simulink model "BruceMotor"  (R2024b)
settings: Solver=VariableStepAuto  StartTime=0.0  StopTime=2  RelTol=1e-3
InitFcn:
  | MotorSimulationParams
values from neighbouring files (symbols this model uses):
  B_PMSM = 0    [MotorSimulationParams.m]
  F_PMSM = 1e-3    (= 0.001)    [MotorSimulationParams.m]
  Id_D = 0    [MotorSimulationParams.m]
  Id_I = 0    [MotorSimulationParams.m]
  Id_P = 10    [MotorSimulationParams.m]
  Id_ref = 0    [MotorSimulationParams.m]
  Iq_D = 0    [MotorSimulationParams.m]
  Iq_I = 0    [MotorSimulationParams.m]
  Iq_P = 100    [MotorSimulationParams.m]
  J_PMSM = 1.879e-6    (= 1.879e-06)    [MotorSimulationParams.m]
  Load_Torque = 0    [MotorSimulationParams.m]
  Pole_Pairs = 1    [MotorSimulationParams.m]
  Ref_Torque = 1e-5    (= 1e-05)    [MotorSimulationParams.m]
  Rline = 1e-3    (= 0.001)    [MotorSimulationParams.m]
  Rs = 312e-3    (= 0.312)    [MotorSimulationParams.m]
  Speed_D = 0    [MotorSimulationParams.m]
  Speed_I = 0    [MotorSimulationParams.m]
  Speed_P = 100    [MotorSimulationParams.m]
  Speed_Ref = Wrated    (= 282.743338823)    [MotorSimulationParams.m]
  Tstep = 5e-6    (= 5e-06)    [MotorSimulationParams.m]
libraries: spsHalfBridgeConverterLib x3, spsdq0toabcLib x2, spsDCVoltageSourceLib x1, spsPermanentMagnetSynchronousMachineLib x1, simulink x1, spsThreePhaseParallelRLCBranchLib x1, spsabctodq0Lib x1, spspowerguiLib x1
settings Model: Creator=pickl  LastModifiedBy=pickl
settings SolverCC: ZeroCrossAlgorithm=Adaptive
settings DebuggingCC: MaskedZcDiagnostic=none  IgnoredZcDiagnostic=none

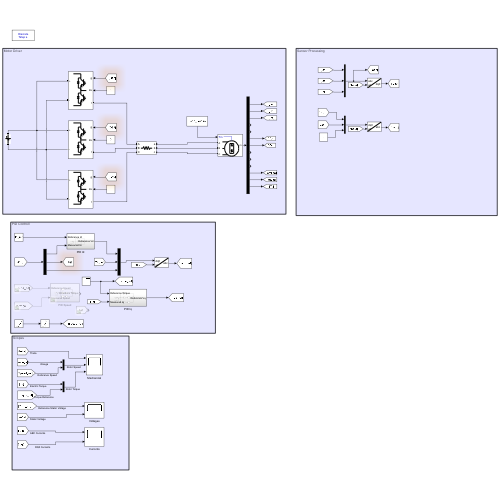
[thumbnail: Simulink's stored preview of the top-level diagram]
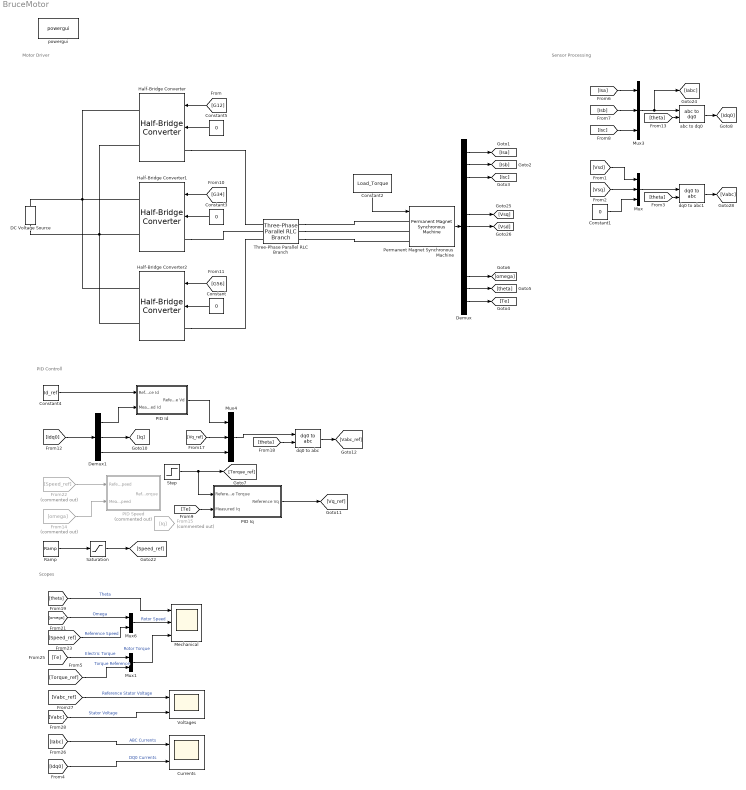
== system BruceMotor ==
  note: Scopes
  note: PID Controll
  note: Sensor Processing
  note: Motor Driver
  Constant{,1,3,5} (4 alike) : Constant  Value=0
  Constant2 : Constant  Value=Load_Torque
  Constant4 : Constant  Value=Id_ref
  Currents : Scope  NumInputPorts=2
  DC Voltage Source : spsDCVoltageSourceLib/DC Voltage Source  Amplitude=10  Measurements=None
  Demux : Demux  Outputs=13
  Demux1 : Demux  Outputs=3
  From14 : From  Commented=on  GotoTag=omega
  From15 : From  Commented=on  GotoTag=Iq
  From22 : From  Commented=on  GotoTag=Speed_ref
  Half-Bridge Converter : spsHalfBridgeConverterLib/Half-Bridge Converter  ModelType=Switching devices  Ron=1e-3  Rs=1e6  Cs=inf  Vforward=[0,0]  Ron_Diode=1e-3  Rs_Diode=1e6  Cs_Diode=inf  Vf_Diode=1e-3  Rs_CurrentSource=inf  Ron_ACsource=1e-3
      settings: LibrarySourceBlock=sps_lib/Power Electronics/Half-Bridge Converter
  Half-Bridge Converter1 : spsHalfBridgeConverterLib/Half-Bridge Converter  ModelType=Switching devices  Ron=1e-3  Rs=1e6  Cs=inf  Vforward=[0,0]  Ron_Diode=1e-3  Rs_Diode=1e6  Cs_Diode=inf  Vf_Diode=1e-3  Rs_CurrentSource=inf  Ron_ACsource=1e-3
      settings: LibrarySourceBlock=sps_lib/Power Electronics/Half-Bridge Converter
  Half-Bridge Converter2 : spsHalfBridgeConverterLib/Half-Bridge Converter  ModelType=Switching devices  Ron=1e-3  Rs=1e6  Cs=inf  Vforward=[0,0]  Ron_Diode=1e-3  Rs_Diode=1e6  Cs_Diode=inf  Vf_Diode=1e-3  Rs_CurrentSource=inf  Ron_ACsource=1e-3
      settings: LibrarySourceBlock=sps_lib/Power Electronics/Half-Bridge Converter
  Mechanical : Scope  NumInputPorts=3
  Mux : Mux  Inputs=3
  Mux1 : Mux  Inputs=2
  Mux3 : Mux  Inputs=3
  Mux4 : Mux  Inputs=3
  Mux6 : Mux  Inputs=2
  PID Id : Subsystem
  PID Iq : Subsystem
  PID Speed : Subsystem  Commented=on
  Permanent Magnet Synchronous Machine : spsPermanentMagnetSynchronousMachineLib/Permanent Magnet Synchronous Machine  NbPhases=3  FluxDistribution=Sinusoidal  RotorType=Round  MechanicalLoad=Torque Tm  PresetModel=No  ShowDetailedParameters=on  MeasurementBus=off  Resistance=Rs  Inductance=8.5e-3  dqInductances=[8.5e-3,8.5e-3]  La=Lq  MachineConstant=Voltage Constant (V_peak L-L / krpm)  Flux=0.0091888  VoltageCst=Kv  TorqueCst=0.04135  Flat=120  Mechanical=[J_PMSM, F_PMSM, Pole_Pairs, B_PMSM]  PolePairs=4  InitialConditions=[0,0, 0,0]  InitialConditions5ph=[0 0 0 0 0 0]  RefAngle=Aligned with phase A axis (original Park)  IterativeDiscreteModel=Trapezoidal non iterative  TsBlock=-1  TsPowergui=0
  Ramp : simulink/Sources/Ramp  slope=Wrated/Tramp  start=0.5  InitialOutput=0
  Saturation : Saturate  UpperLimit=Speed_Ref  LowerLimit=-Speed_Ref
  Step : Step  Time=0.2  After=Ref_Torque  SampleTime=0
  Three-Phase Parallel RLC Branch : spsThreePhaseParallelRLCBranchLib/Three-Phase Parallel RLC Branch  LConnTagsString=A|B|C  RConnTagsString=A|B|C  BranchType=R  Resistance=Rline  Inductance=1e-3  Capacitance=1e-6  Measurements=None
  Voltages : Scope  NumInputPorts=2
  abc to dq0 : spsabctodq0Lib/abc to dq0  Alignment=Aligned with phase A axis
  dq0 to abc : spsdq0toabcLib/dq0 to abc  Alignment=Aligned with phase A axis
  dq0 to abc1 : spsdq0toabcLib/dq0 to abc  Alignment=Aligned with phase A axis
  powergui : spspowerguiLib/powergui  Priority=1  SimulationMode=Discrete  SampleTime=Tstep  frequency=60  Iterations=50  frequencyindice=0  Pbase=100e6  ErrMax=1e-4  UnitsV=kV  UnitsW=MW  buscounter=0  FunctionMessages=off  echomessages=off  EnableUseOfTLC=off  CurrentSourceSwitches=off  DisableSnubberDevices=off  DisableRonSwitches=off  DisableVfSwitches=off  DisplayEquations=off  AutomaticDiscreteSolvers=off  SolverType=Tustin/Backward Euler (TBE)  Interpol=off  ExternalGateDelay=off  methode=off  Ts=100  x0status=zero  SPID=on  SwTol=0  HookPort=off  NonlinearTolerance=1e-4  nMaxIteration=100  ContinueOnMaxIteration=off  RestoreLinks=warning  ResistiveCurrentMeasurement=off  Frange=[0:2:500]  Ylog=off  Xlog=on  ShowGrid=off  save=off  variable=ZData  structure=0  ZoomFFT=off  StartTime=0.0  cycles=1  DisplayStyle=1  fundamental=60  FreqAxis=off  MaxFrequency=1000  frequencyindicesteady=1  RmsSteady=1  display=off
  wires:
  Permanent Magnet Synchronous Machine/1 -> Demux/1
  Demux/1 -> [Isa]
  Demux/2 -> [Isb]
  Demux/3 -> [Isc]
  [Isa] -> Mux3/1
  [Isb] -> Mux3/2
  [Isc] -> Mux3/3
  Mux3/1 -> [Iabc], abc to dq0/1
  abc to dq0/1 -> [Idq0]
  [Idq0] -> Demux1/1
  Demux1/3 -> Mux4/3
  Demux1/2 -> [Iq]
  [Vq_ref] -> Mux4/2
  Mux4/1 -> dq0 to abc/1
  [theta] -> abc to dq0/2
  [theta] -> dq0 to abc/2
  dq0 to abc/1 -> [Vabc_ref]
  [theta] -> Mechanical/1  "Theta"
  [omega] -> Mux6/1  "Omega"
  [Speed_ref] -> Mux6/2  "Reference Speed"
  Mux6/1 -> Mechanical/2  "Rotor Speed"
  Ramp/1 -> Saturation/1
  Saturation/1 -> [Speed_ref]
  [Vsd] -> Mux/1
  [Vsq] -> Mux/2
  Constant1/1 -> Mux/3
  Demux/6 -> [Vsq]
  Demux/7 -> [Vsd]
  Demux/13 -> [Te]
  Demux/12 -> [theta]
  Demux/11 -> [omega]
  Mux/1 -> dq0 to abc1/1
  dq0 to abc1/1 -> [Vabc]
  [theta] -> dq0 to abc1/2
  Constant2/1 -> Permanent Magnet Synchronous Machine/1
  PID Iq/1(Reference Vq) -> [Vq_ref]
  From22/1 -> PID Speed/1(Reference Speed)
  From14/1 -> PID Speed/2(Measured Speed)
  Demux1/1 -> PID Id/2(Measured Id)
  Constant4/1 -> PID Id/1(Reference Id)
  PID Id/1(Reference Vd) -> Mux4/1
  [Vabc_ref] -> Voltages/1  "Reference Stator Voltage"
  [Vabc] -> Voltages/2  "Stator Voltage"
  [Iabc] -> Currents/1  "ABC Currents"
  [Idq0] -> Currents/2  "DQ0 Currents"
  Step/1 -> PID Iq/1(Reference Torque), [Torque_ref]
  [Te] -> Mux1/1  "Electric Torque"
  [Torque_ref] -> Mux1/2  "Torque Reference"
  Mux1/1 -> Mechanical/3  "Rotor Torque"
  [Te] -> PID Iq/2(Measured Iq)
  [G34] -> Half-Bridge Converter1/1
  Constant/1 -> Half-Bridge Converter2/2
  [G56] -> Half-Bridge Converter2/1
  [G12] -> Half-Bridge Converter/1
  Constant3/1 -> Half-Bridge Converter1/2
  Constant5/1 -> Half-Bridge Converter/2
  connections:
  Three-Phase Parallel RLC Branch/RConn2 -- Permanent Magnet Synchronous Machine/LConn2
  Three-Phase Parallel RLC Branch/RConn1 -- Permanent Magnet Synchronous Machine/LConn1
  Three-Phase Parallel RLC Branch/RConn3 -- Permanent Magnet Synchronous Machine/LConn3
  Half-Bridge Converter1/RConn1 -- DC Voltage Source/RConn1 -- Half-Bridge Converter2/RConn1 -- Half-Bridge Converter/RConn1
  DC Voltage Source/LConn1 -- Half-Bridge Converter/RConn2 -- Half-Bridge Converter2/RConn2 -- Half-Bridge Converter1/RConn2
  Half-Bridge Converter/LConn1 -- Three-Phase Parallel RLC Branch/LConn1
  Half-Bridge Converter1/LConn1 -- Three-Phase Parallel RLC Branch/LConn2
  Half-Bridge Converter2/LConn1 -- Three-Phase Parallel RLC Branch/LConn3

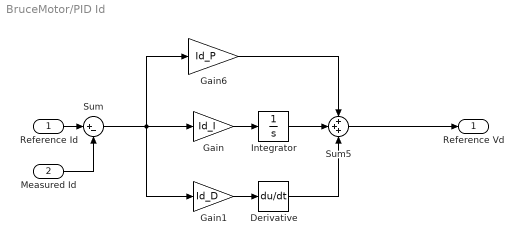
== system BruceMotor/PID Id ==
  Reference Id : Inport
  Measured Id : Inport  Port=2
  Derivative : Derivative
  Gain : Gain  Gain=Id_I
  Gain1 : Gain  Gain=Id_D
  Gain6 : Gain  Gain=Id_P
  Integrator : Integrator
  Sum : Sum  Inputs=|+-
  Sum5 : Sum  Inputs=+++
  Reference Vd : Outport
  wires:
  Reference Id/1 -> Sum/1
  Measured Id/1 -> Sum/2
  Gain/1 -> Integrator/1
  Gain6/1 -> Sum5/1
  Sum/1 -> Gain1/1, Gain6/1, Gain/1
  Gain1/1 -> Derivative/1
  Sum5/1 -> Reference Vd/1
  Integrator/1 -> Sum5/2
  Derivative/1 -> Sum5/3

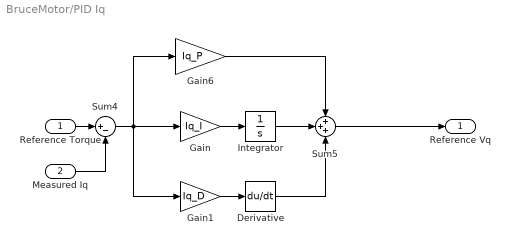
== system BruceMotor/PID Iq ==
  Reference Torque : Inport
  Measured Iq : Inport  Port=2
  Derivative : Derivative
  Gain : Gain  Gain=Iq_I
  Gain1 : Gain  Gain=Iq_D
  Gain6 : Gain  Gain=Iq_P
  Integrator : Integrator
  Sum4 : Sum  Inputs=|+-
  Sum5 : Sum  Inputs=+++
  Reference Vq : Outport
  wires:
  Measured Iq/1 -> Sum4/2
  Derivative/1 -> Sum5/3
  Gain/1 -> Integrator/1
  Sum4/1 -> Gain1/1, Gain6/1, Gain/1
  Gain6/1 -> Sum5/1
  Reference Torque/1 -> Sum4/1
  Sum5/1 -> Reference Vq/1
  Integrator/1 -> Sum5/2
  Gain1/1 -> Derivative/1

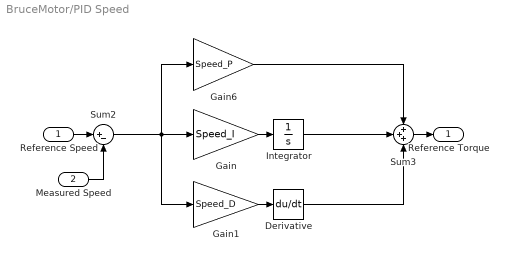
== system BruceMotor/PID Speed ==
  Reference Speed : Inport
  Measured Speed : Inport  Port=2
  Derivative : Derivative
  Gain : Gain  Gain=Speed_I
  Gain1 : Gain  Gain=Speed_D
  Gain6 : Gain  Gain=Speed_P
  Integrator : Integrator
  Sum2 : Sum  Inputs=|+-
  Sum3 : Sum  Inputs=+++
  Reference Torque : Outport
  wires:
  Sum3/1 -> Reference Torque/1
  Derivative/1 -> Sum3/3
  Integrator/1 -> Sum3/2
  Gain6/1 -> Sum3/1
  Reference Speed/1 -> Sum2/1
  Measured Speed/1 -> Sum2/2
  Gain/1 -> Integrator/1
  Sum2/1 -> Gain1/1, Gain/1, Gain6/1
  Gain1/1 -> Derivative/1
